simulink model "Assignment_TestGen16"  (R2017b)
settings: Solver=FixedStepDiscrete  StartTime=0.0  StopTime=10.0  RelTol=1e-3
undefined symbols (not defined in the file): Block_TestLib, enable_trigger
settings Model: Creator=hbourbou  LastModifiedBy=hbourbou
settings DebuggingCC: ParameterOverflowMsg=none

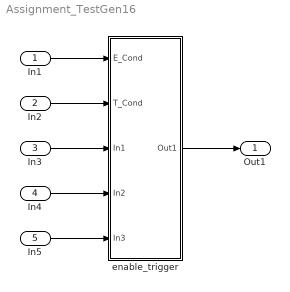
== system Assignment_TestGen16 ==
  In1 : Inport
  In2 : Inport  Port=2
  In3 : Inport  Port=3
  In4 : Inport  Port=4
  In5 : Inport  Port=5
  enable_trigger : Subsystem  AncestorBlock=Block_TestLib/enable_trigger
  Out1 : Outport
  wires:
  In1/1 -> enable_trigger/1(E_Cond)
  In2/1 -> enable_trigger/2(T_Cond)
  In3/1 -> enable_trigger/3(In1)
  In4/1 -> enable_trigger/4(In2)
  In5/1 -> enable_trigger/5(In3)
  enable_trigger/1(Out1) -> Out1/1

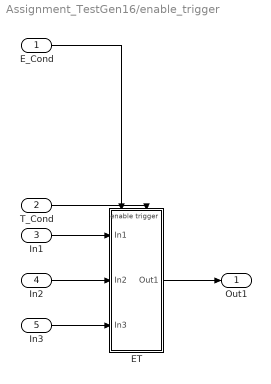
== system Assignment_TestGen16/enable_trigger ==
  E_Cond : Inport  OutDataTypeStr=boolean
  T_Cond : Inport  Port=2  OutDataTypeStr=boolean
  In1 : Inport  Port=3
  In2 : Inport  Port=4
  In3 : Inport  Port=5
  ET : Subsystem  TreatAsAtomicUnit=on
  Out1 : Outport
  wires:
  T_Cond/1 -> ET/Trigger
  E_Cond/1 -> ET/Enable
  In1/1 -> ET/1(In1)
  In2/1 -> ET/2(In2)
  In3/1 -> ET/3(In3)
  ET/1(Out1) -> Out1/1

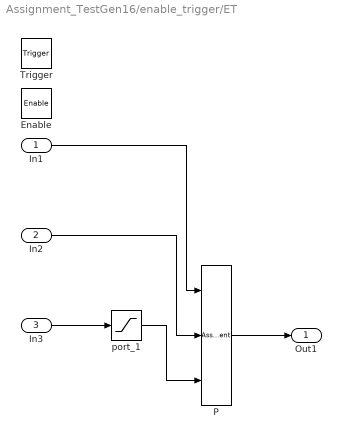
== system Assignment_TestGen16/enable_trigger/ET ==
  In1 : Inport  OutDataTypeStr=double  PortDimensions=[3 3 3 3]
  In2 : Inport  Port=2  OutDataTypeStr=double  PortDimensions=[3 2 2 2]
  In3 : Inport  Port=3  OutMin=0  OutMax=1
  Enable : EnablePort
  Trigger : TriggerPort  VariantControl=Variant
  P : Assignment  NumberOfDimensions=4  IndexMode=Zero-based  DiagnosticForDimensions=Warning  IndexOptions=Assign all,Index vector (dialog),Index vector (port),Starting index (dialog)  Indices=[],[1,2],[],1  OutputSizes=,,,
  port_1 : Saturate  UpperLimit=1  LowerLimit=0
  Out1 : Outport
  wires:
  In1/1 -> P/1
  In2/1 -> P/2
  port_1/1 -> P/3
  In3/1 -> port_1/1
  P/1 -> Out1/1
